simulink model "sampleModel1885"  (R2023a)
settings: Solver=VariableStepAuto  StartTime=0.0  StopTime=10.0  RelTol=1e-3
libraries: hdlsllib x5
settings Model: Creator=user1  LastModifiedBy=user1

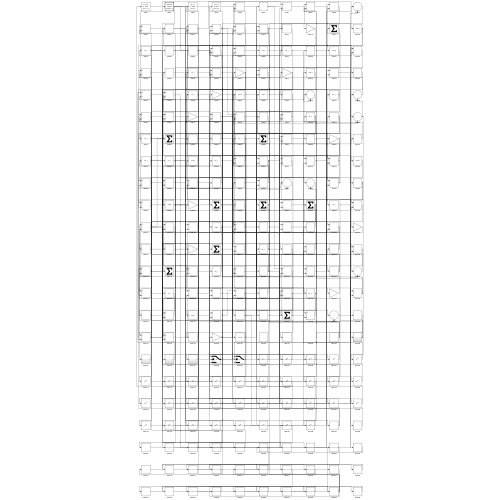
[thumbnail: Simulink's stored preview of the top-level diagram]
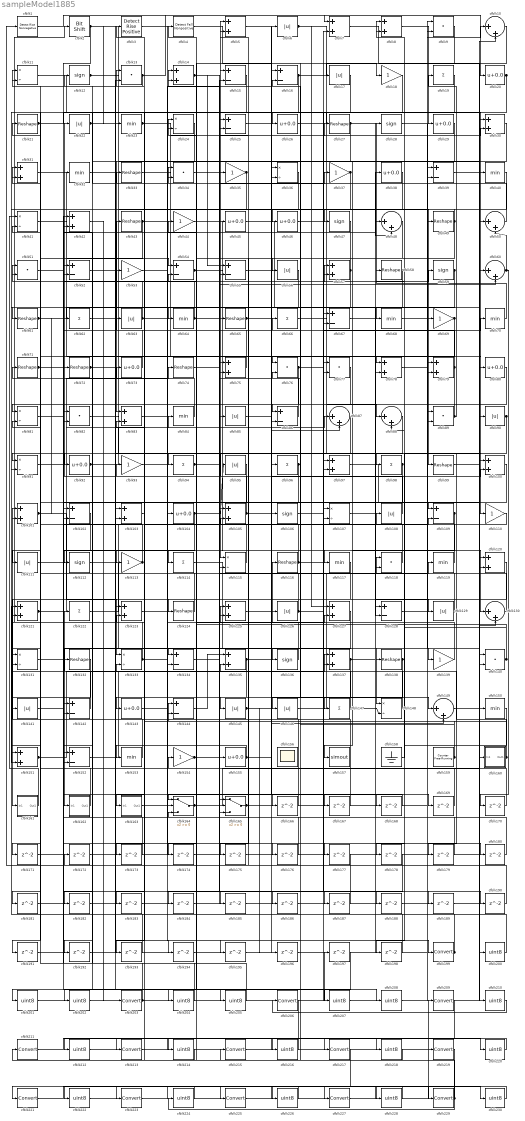
== system sampleModel1885 ==
  cfblk1 : hdlsllib/Logic and Bit Operations/Detect Rise Nonnegative  vinit=0  OutDataTypeStr=boolean
  cfblk{10,48,50,60,87..88,130,149} (8 alike) : Sum  Inputs=|++
  cfblk{5,7..8,14,30..31,42,57,75,78..79,83,97,100..101,103,105,120..121,123,125,127,135,137,151} (25 alike) : Sum
  cfblk{15..16,25,39,52,54..55,67,86,102,109,128,134,142,144,152} (16 alike) : Sum  Inputs=+-
  cfblk{20,26,29,38,45..46,73,80,92,104,143,155} (12 alike) : Bias  Bias=0.0  SaturateOnIntegerOverflow=off
  cfblk{12,28,47,59,106,112,136} (7 alike) : Signum
  cfblk{11,24,36,41,81,91,107,115,131,133,148} (11 alike) : Product  Inputs=*/  RndMeth=Zero  SaturateOnIntegerOverflow=on
  cfblk{6,17,22,56,63,85,90,95,108,111,126,129,141,145..146} (15 alike) : Abs  SaturateOnIntegerOverflow=off
  cfblk{18,35,37,44,53,69,93,110,113,139,154} (11 alike) : Gain
  cfblk{19,62,66,94,96,98,114,122,147} (9 alike) : Sum  Inputs=+
  cfblk{21,27,33,43,49,58,61,65,71..72,74,99,116,124,132,138} (16 alike) : Reshape
  cfblk{23,32,40,64,68,70,84,117,119,150,153} (11 alike) : MinMax
  cfblk{9,13,34,51,76..77,82,89,118,140} (10 alike) : DotProduct  OutDataTypeStr=Inherit: Inherit via internal rule
  cfblk156 : Scope
      settings: Floating=on
  cfblk157 : ToWorkspace  VariableName=simout  SaveFormat=Timeseries  SampleTime=-1
  cfblk158 : Ground
  cfblk159 : hdlsllib/Sources/Counter Free-Running  NumBits=16  tsamp=-1
  cfblk160 : Subsystem
      settings: LibrarySourceBlock=|
      | hdlsllib/Ports &
      | Subsystems/Subsystem
  cfblk161 : Subsystem
      settings: LibrarySourceBlock=|
      | hdlsllib/Ports &
      | Subsystems/Subsystem
  cfblk162 : Subsystem
      settings: LibrarySourceBlock=|
      | hdlsllib/Ports &
      | Subsystems/Subsystem
  cfblk163 : Subsystem
      settings: LibrarySourceBlock=|
      | hdlsllib/Ports &
      | Subsystems/Subsystem
  cfblk164 : Switch  SaturateOnIntegerOverflow=off  InputSameDT=off
  cfblk165 : Switch  SaturateOnIntegerOverflow=off  InputSameDT=off
  cfblk{166..198} (33 alike) : Delay  SampleTime=1
  cfblk{199,203,206,209,211,213,215,217,219,221,223,225,227,229} (14 alike) : DataTypeConversion  SaturateOnIntegerOverflow=off  RndMeth=Floor
  cfblk2 : hdlsllib/Logic and Bit Operations/Bit Shift  mode=Shift Left Logical  N=0
  cfblk{200..202,204..205,207..208,210,212,214,216,218,220,222,224,226,228,230} (18 alike) : DataTypeConversion  OutDataTypeStr=uint8  SaturateOnIntegerOverflow=off  RndMeth=Floor
  cfblk3 : hdlsllib/Logic and Bit Operations/Detect Rise Positive  vinit=0  OutDataTypeStr=boolean
  cfblk4 : hdlsllib/Logic and Bit Operations/Detect Fall Nonpositive  vinit=0  OutDataTypeStr=boolean
  wires:
  cfblk62/1 -> cfblk94/1
  cfblk105/1 -> cfblk5/1, cfblk149/2
  cfblk110/1 -> cfblk14/1
  cfblk121/1 -> cfblk74/1, cfblk208/1
  cfblk87/1 -> cfblk115/1
  cfblk27/1 -> cfblk83/1, cfblk48/2
  cfblk133/1 -> cfblk2/1, cfblk125/1
  cfblk108/1 -> cfblk22/1
  cfblk26/1 -> cfblk110/1
  cfblk86/1 -> cfblk35/1
  cfblk44/1 -> cfblk76/1
  cfblk6/1 -> cfblk88/1, cfblk127/1
  cfblk16/1 -> cfblk18/1, cfblk14/2, cfblk91/2
  cfblk34/1 -> cfblk100/1
  cfblk70/1 -> cfblk28/1
  cfblk88/1 -> cfblk91/1
  cfblk144/1 -> cfblk135/1
  cfblk12/1 -> cfblk80/1, cfblk194/1
  cfblk89/1 -> cfblk81/1, cfblk19/1
  cfblk153/1 -> cfblk101/1
  cfblk54/1 -> cfblk130/1, cfblk67/2
  cfblk130/1 -> cfblk75/1
  cfblk113/1 -> cfblk21/1, cfblk81/2
  cfblk60/1 -> cfblk50/2, cfblk170/1
  cfblk134/1 -> cfblk37/1
  cfblk13/1 -> cfblk20/1, cfblk11/2
  cfblk136/1 -> cfblk4/1
  cfblk92/1 -> cfblk84/1, cfblk87/1, cfblk205/1
  cfblk45/1 -> cfblk99/1
  cfblk161/1(Out1) -> cfblk41/1
  cfblk148/1 -> cfblk122/1
  cfblk120/1 -> cfblk161/1(In1)
  cfblk29/1 -> cfblk124/1
  cfblk116/1 -> cfblk73/1, cfblk188/1
  cfblk11/1 -> cfblk40/1
  cfblk61/1 -> cfblk68/1, cfblk207/1
  cfblk122/1 -> cfblk108/1
  cfblk139/1 -> cfblk116/1
  cfblk73/1 -> cfblk43/1
  cfblk140/1 -> cfblk24/1, cfblk8/2
  cfblk98/1 -> cfblk145/1, cfblk111/1
  cfblk43/1 -> cfblk151/1, cfblk180/1
  cfblk111/1 -> cfblk117/1
  cfblk114/1 -> cfblk139/1
  cfblk74/1 -> cfblk155/1
  cfblk109/1 -> cfblk157/1, cfblk105/2
  cfblk107/1 -> cfblk129/1
  cfblk142/1 -> cfblk101/2
  cfblk66/1 -> cfblk150/1
  cfblk23/1 -> cfblk107/1, cfblk30/2
  cfblk8/1 -> cfblk29/1
  cfblk101/1 -> cfblk133/1, cfblk62/1, cfblk109/2
  cfblk31/1 -> cfblk78/1
  cfblk72/1 -> cfblk57/1, cfblk98/1
  cfblk65/1 -> cfblk149/1, cfblk175/1
  cfblk5/1 -> cfblk106/1
  cfblk17/1 -> cfblk63/1
  cfblk22/1 -> cfblk89/1, cfblk189/1
  cfblk30/1 -> cfblk47/1
  cfblk118/1 -> cfblk33/1
  cfblk149/1 -> cfblk30/1
  cfblk104/1 -> cfblk95/1, cfblk182/1
  cfblk58/1 -> cfblk64/1, cfblk131/2
  cfblk93/1 -> cfblk15/1
  cfblk59/1 -> cfblk128/2, cfblk125/2
  cfblk14/1 -> cfblk55/1, cfblk177/1
  cfblk10/1 -> cfblk134/1
  cfblk19/1 -> cfblk107/2
  cfblk154/1 -> cfblk25/1, cfblk127/2
  cfblk124/1 -> cfblk72/1
  cfblk28/1 -> cfblk69/1
  cfblk112/1 -> cfblk148/1
  cfblk40/1 -> cfblk113/1
  cfblk7/1 -> cfblk160/1(In1)
  cfblk146/1 -> cfblk38/1
  cfblk46/1 -> cfblk57/2
  cfblk160/1(Out1) -> cfblk144/1, cfblk135/2
  cfblk97/1 -> cfblk120/1
  cfblk83/1 -> cfblk104/1
  cfblk126/1 -> cfblk25/2, cfblk13/1, cfblk168/1
  cfblk1/1 -> cfblk7/1
  cfblk36/1 -> cfblk102/2
  cfblk50/1 -> cfblk12/1
  cfblk152/1 -> cfblk17/1
  cfblk127/1 -> cfblk162/1(In1)
  cfblk91/1 -> cfblk15/2
  cfblk20/1 -> cfblk136/1, cfblk34/2
  cfblk159/1 -> cfblk93/1, cfblk88/2, cfblk76/2
  cfblk151/1 -> cfblk137/1, cfblk55/2, cfblk71/1
  cfblk15/1 -> cfblk61/1
  cfblk106/1 -> cfblk138/1
  cfblk76/1 -> cfblk132/1, cfblk70/1, cfblk191/1
  cfblk138/1 -> cfblk58/1, cfblk184/1
  cfblk21/1 -> cfblk26/1, cfblk114/1, cfblk109/1
  cfblk35/1 -> cfblk152/1, cfblk165/3
  cfblk48/1 -> cfblk105/1
  cfblk69/1 -> cfblk141/1, cfblk165/2
  cfblk49/1 -> cfblk115/2, cfblk46/1
  cfblk52/1 -> cfblk123/1
  cfblk75/1 -> cfblk32/1
  cfblk162/1(Out1) -> cfblk31/1
  cfblk90/1 -> cfblk178/1, cfblk179/1
  cfblk129/1 -> cfblk11/1, cfblk51/2
  cfblk96/1 -> cfblk16/2, cfblk131/1
  cfblk164/1 -> cfblk130/2, cfblk118/1
  cfblk53/1 -> cfblk199/1
  cfblk100/1 -> cfblk163/1(In1)
  cfblk141/1 -> cfblk45/1
  cfblk115/1 -> cfblk44/1
  cfblk128/1 -> cfblk10/1
  cfblk158/1 -> cfblk8/1
  cfblk155/1 -> cfblk36/1, cfblk153/1
  cfblk4/1 -> cfblk96/1
  cfblk137/1 -> cfblk119/1, cfblk183/1
  cfblk78/1 -> cfblk49/1
  cfblk102/1 -> cfblk142/2
  cfblk9/1 -> cfblk146/1
  cfblk165/1 -> cfblk65/1, cfblk9/1
  cfblk33/1 -> cfblk97/2
  cfblk2/1 -> cfblk60/1, cfblk24/2, cfblk152/2, cfblk23/1, cfblk195/1
  cfblk68/1 -> cfblk140/2
  cfblk143/1 -> cfblk59/1
  cfblk84/1 -> cfblk51/1
  cfblk41/1 -> cfblk54/1
  cfblk94/1 -> cfblk27/1, cfblk60/2
  cfblk63/1 -> cfblk31/2, cfblk75/2
  cfblk64/1 -> cfblk52/1, cfblk186/1
  cfblk85/1 -> cfblk126/1
  cfblk82/1 -> cfblk85/1
  cfblk135/1 -> cfblk164/1, cfblk87/2
  cfblk71/1 -> cfblk48/1, cfblk137/2
  cfblk80/1 -> cfblk86/1
  cfblk37/1 -> cfblk82/2, cfblk151/2
  cfblk42/1 -> cfblk203/1
  cfblk147/1 -> cfblk148/2, cfblk34/1
  cfblk57/1 -> cfblk56/1, cfblk192/1
  cfblk125/1 -> cfblk6/1
  cfblk24/1 -> cfblk112/1
  cfblk79/1 -> cfblk143/1, cfblk52/2
  cfblk103/1 -> cfblk3/1
  cfblk55/1 -> cfblk90/1
  cfblk18/1 -> cfblk92/1
  cfblk145/1 -> cfblk100/2, cfblk196/1
  cfblk119/1 -> cfblk83/2
  cfblk67/1 -> cfblk79/1
  cfblk38/1 -> cfblk147/1
  cfblk32/1 -> cfblk103/2
  cfblk3/1 -> cfblk166/1
  cfblk166/1 -> cfblk103/1
  cfblk25/1 -> cfblk167/1
  cfblk167/1 -> cfblk41/2
  cfblk168/1 -> cfblk164/2
  cfblk51/1 -> cfblk169/1
  cfblk169/1 -> cfblk82/1
  cfblk170/1 -> cfblk128/1
  cfblk132/1 -> cfblk171/1
  cfblk171/1 -> cfblk78/2
  cfblk172/1 -> cfblk134/2
  cfblk77/1 -> cfblk173/1
  cfblk173/1 -> cfblk142/1
  cfblk47/1 -> cfblk174/1
  cfblk174/1 -> cfblk144/2
  cfblk175/1 -> cfblk50/1
  cfblk81/1 -> cfblk176/1
  cfblk176/1 -> cfblk16/1
  cfblk177/1 -> cfblk1/1
  cfblk179/1 -> cfblk54/2
  cfblk180/1 -> cfblk102/1
  cfblk95/1 -> cfblk181/1
  cfblk181/1 -> cfblk165/1
  cfblk182/1 -> cfblk7/2
  cfblk183/1 -> cfblk86/2
  cfblk184/1 -> cfblk89/2
  cfblk123/1 -> cfblk185/1
  cfblk185/1 -> cfblk120/2
  cfblk186/1 -> cfblk67/1
  cfblk131/1 -> cfblk187/1
  cfblk187/1 -> cfblk5/2
  cfblk188/1 -> cfblk9/2
  cfblk189/1 -> cfblk10/2
  cfblk163/1(Out1) -> cfblk190/1
  cfblk190/1 -> cfblk97/1
  cfblk191/1 -> cfblk13/2
  cfblk192/1 -> cfblk36/2
  cfblk56/1 -> cfblk193/1
  cfblk193/1 -> cfblk121/1
  cfblk194/1 -> cfblk164/3
  cfblk195/1 -> cfblk118/2
  cfblk196/1 -> cfblk79/2
  cfblk150/1 -> cfblk198/1
  cfblk198/1 -> cfblk133/2
  cfblk199/1 -> cfblk172/1, cfblk77/1
  cfblk99/1 -> cfblk200/1
  cfblk200/1 -> cfblk53/1
  cfblk197/1 -> cfblk201/1
  cfblk201/1 -> cfblk140/1
  cfblk117/1 -> cfblk202/1
  cfblk202/1 -> cfblk197/1
  cfblk203/1 -> cfblk77/2, cfblk121/2
  cfblk178/1 -> cfblk204/1
  cfblk204/1 -> cfblk42/1
  cfblk205/1 -> cfblk42/2
  cfblk207/1 -> cfblk39/1
  cfblk208/1 -> cfblk39/2
  cfblk39/1 -> cfblk210/1
  cfblk210/1 -> cfblk206/1
  cfblk206/1 -> cfblk212/1
  cfblk212/1 -> cfblk209/1
  cfblk209/1 -> cfblk214/1
  cfblk214/1 -> cfblk211/1
  cfblk211/1 -> cfblk216/1
  cfblk216/1 -> cfblk213/1
  cfblk213/1 -> cfblk218/1
  cfblk218/1 -> cfblk215/1
  cfblk215/1 -> cfblk220/1
  cfblk220/1 -> cfblk217/1
  cfblk217/1 -> cfblk222/1
  cfblk222/1 -> cfblk219/1
  cfblk219/1 -> cfblk224/1
  cfblk224/1 -> cfblk221/1
  cfblk221/1 -> cfblk226/1
  cfblk226/1 -> cfblk223/1
  cfblk227/1 -> cfblk229/1
  cfblk223/1 -> cfblk228/1
  cfblk228/1 -> cfblk225/1
  cfblk229/1 -> cfblk66/1, cfblk154/1, cfblk123/2
  cfblk225/1 -> cfblk230/1
  cfblk230/1 -> cfblk227/1

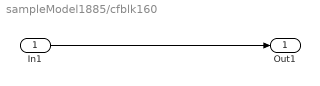
== system sampleModel1885/cfblk160 ==
  In1 : Inport
  Out1 : Outport
  wires:
  In1/1 -> Out1/1

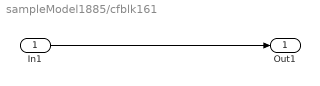
== system sampleModel1885/cfblk161 ==
  In1 : Inport
  Out1 : Outport
  wires:
  In1/1 -> Out1/1

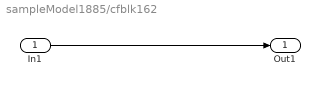
== system sampleModel1885/cfblk162 ==
  In1 : Inport
  Out1 : Outport
  wires:
  In1/1 -> Out1/1

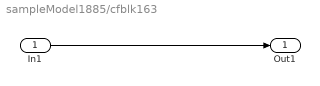
== system sampleModel1885/cfblk163 ==
  In1 : Inport
  Out1 : Outport
  wires:
  In1/1 -> Out1/1
